simulink model "testmiei"  (R2020b)
settings: Solver=VariableStepAuto  StartTime=0.0  StopTime=1  RelTol=1e-3
values from neighbouring files (symbols this model uses):
  A = [0 1 ... (first row only)    [TestDIST_EFFECT_DCmotor_zp(1).m]    (also in TestDIST_EFFECT_DCmotor_zp.m; lqr_DOB_2_5.mat = [0  1; 0  0]; lqr_DOB_5.mat = [0  1; 0  0]; lqr_DOB_8.mat = [0  1; 0  0])
  B = [0; Kt/Rm/Jt]    [TestDIST_EFFECT_DCmotor_zp(1).m]    (also in TestDIST_EFFECT_DCmotor_zp.m; lqr_DOB_2_5.mat = [0 239.250934036]; lqr_DOB_5.mat = [0 239.250934036]; lqr_DOB_8.mat = [0 239.250934036])
  KK = dlqr(Fs,Gs,Q,R)    [TestDIST_EFFECT_DCmotor_zp(1).m]    (also in TestDIST_EFFECT_DCmotor_zp.m; lqr_DOB_2_5.mat = [27.9647466006 0.483496818901]; lqr_DOB_5.mat = [27.9647466006 0.483496818901]; lqr_DOB_8.mat = [27.9647466006 0.483496818901])
  Wz = minreal([1 0]*((eye(2)*z-Fs+Gs*KK))^-1*Gs*KK(1),0.01)    [TestDIST_EFFECT_DCmotor_zp(1).m]    (also in TestDIST_EFFECT_DCmotor_zp.m)
  z = tf('z',Ts)    [TestDIST_EFFECT_DCmotor_zp(1).m]    (also in TestDIST_EFFECT_DCmotor_zp.m)
libraries: cstblocks x1
settings Model: Creator=marco  LastModifiedBy=marco

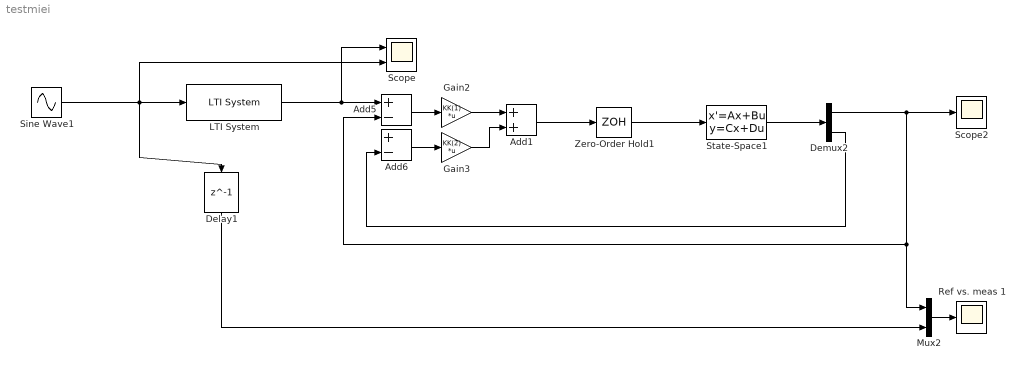
== system testmiei ==
  Add1 : Sum
  Add5 : Sum  Inputs=+-
  Add6 : Sum  Inputs=+-
  Delay1 : Delay  DelayLength=1
  Demux2 : Demux  Outputs=2
  Gain2 : Gain  Gain=KK(1)  Multiplication=Matrix(K*u)
  Gain3 : Gain  Gain=KK(2)  Multiplication=Matrix(K*u)
  LTI System : cstblocks/LTI System  sys=(1/Wz)*z^-1  IC=[]
  Mux2 : Mux  Inputs=2
  Ref vs. meas 1 : Scope
  Scope : Scope  NumInputPorts=2
  Scope2 : Scope
  Sine Wave1 : Sin  SineType=Sample based  Amplitude=0.1  Samples=50  SampleTime=.001
  State-Space1 : StateSpace  A=A(1:2,1:2)  B=B(1:2)  C=eye(2)  D=[0;0]  InitialCondition=0
  Zero-Order Hold1 : ZeroOrderHold  SampleTime=0.001
  wires:
  Gain2/1 -> Add1/1
  Mux2/1 -> Ref vs. meas 1/1
  Gain3/1 -> Add1/2
  Add5/1 -> Gain2/1
  Add6/1 -> Gain3/1
  Demux2/2 -> Add6/2
  Sine Wave1/1 -> LTI System/1, Delay1/1, Scope/2
  LTI System/1 -> Scope/1, Add5/1
  Add1/1 -> Zero-Order Hold1/1
  Delay1/1 -> Mux2/2
  State-Space1/1 -> Demux2/1
  Demux2/1 -> Add5/2, Mux2/1, Scope2/1
  Zero-Order Hold1/1 -> State-Space1/1
